simulink model "test4"  (R2024a)
settings: Solver=FixedStepAuto  StartTime=0.0  StopTime=10  FixedStep=0.001  MaxStep=1e-2  RelTol=1e-3
values from neighbouring files (symbols this model uses):
  Current_Torque_ratio = -10.0    [test4.sldd]
  Sigmoid_Range = 2.0    [test4.sldd]
  Simple_HZ = 10.0    [test4.sldd]
libraries: fl_lib x12, nesl_utility x10, sdl_lib x4, slpidlib x3, simulink x2
settings Model: DataDictionary=test4.sldd  Creator=18311  LastModifiedBy=18311

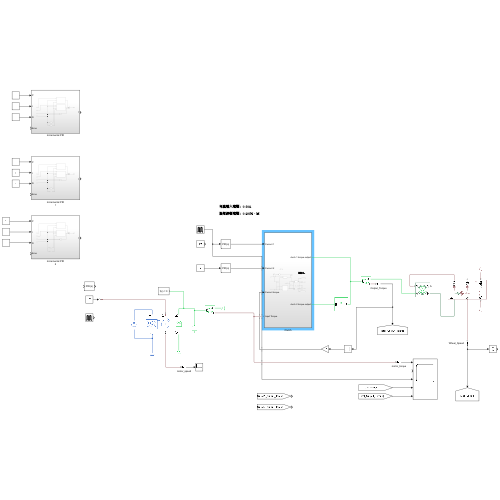
[thumbnail: Simulink's stored preview of the top-level diagram]
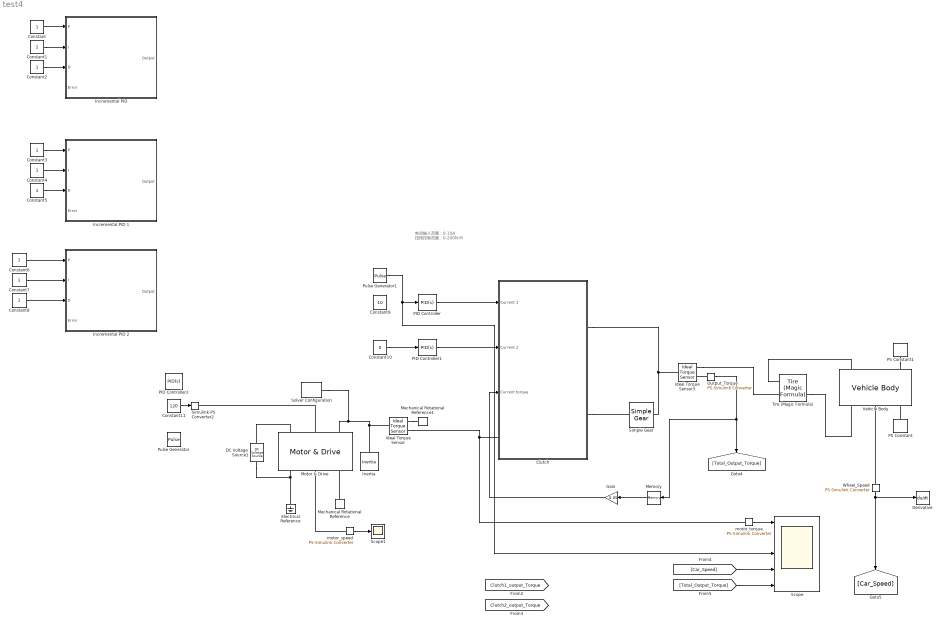
== system test4 ==
  note: 电流输入范围：0-10A
      | 扭矩控制范围：0-200N·M
  Clutch : Subsystem
  Constant{,1..8} (9 alike) : Constant
  Constant10 : Constant  Value=0
  Constant11 : Constant  Value=120
  Constant9 : Constant  Value=10
  DC Voltage Source1 : fl_lib/Electrical/Electrical Sources/DC Voltage Source  v0=220 V
  Derivative : Derivative
  Electrical Reference : fl_lib/Electrical/Electrical Elements/Electrical Reference
  Gain : Gain  Gain=0.05
  Ideal Torque Sensor : fl_lib/Mechanical/Mechanical Sensors/Ideal Torque Sensor
  Ideal Torque Sensor3 : fl_lib/Mechanical/Mechanical Sensors/Ideal Torque Sensor
  "Incremental PID " : Subsystem
  Incremental PID 1 : Subsystem
  Incremental PID 2 : Subsystem
  Inertia : fl_lib/Mechanical/Rotational Elements/Inertia  inertia=0.01 kg*m^2  num_ports=foundation.enum.numPorts2.one  w_specify=off  w_priority=High  w=0 rad/s  w_nominal_specify=off  w_nominal_value=1  w_nominal_unit=rad/s  t_specify=off  t_priority=None  t=0 N*m  t_nominal_specify=off  t_nominal_value=1  t_nominal_unit=N*m
  Mechanical Rotational Reference : fl_lib/Mechanical/Rotational Elements/Mechanical Rotational Reference
  Mechanical Rotational Reference1 : fl_lib/Mechanical/Rotational Elements/Mechanical Rotational Reference
  Memory : Memory
  Motor & Drive : sdl_lib/Engines & Motors/Motor & Drive  torque_max=150 N*m  power_max=20 kW  Tc=1 s  eff=75  w_eff=100 rpm  T_eff=400 N*m  thermal_port=simscape.enum.thermaleffects.omit  thermal_mass=100 J/K  temperature_specify=off  temperature_priority=High  temperature=300 K  temperature_nominal_specify=off  temperature_nominal_value=1  temperature_nominal_unit=K
      settings: InternalSimscapePortConfiguration="{\"Bottom\":[],\"Left\":[{\"id\":\"Vp\",\"label\":\"+\",\"type\":\"foundation.electrical.electrical\"},{\"id\":\"Tr\",\"label\":\"Tr\",\"type\":\"input\"},{\"id\":\"R\",\"label\":\"R\",\"type\":\"foundation.mechanical.rotational.rotational\"}],\"Right\":[{\"id\":\"Vm\",\"label\":\"-\",\"type\":\"foundation.electrical.electrical\"},{\"id\":\"Omega\",\"label\":\"w\",\"type\":\"output\"},{\"id\":\"C\",\"label\":\"C\",\"type\":\"foundation.mechanical.rotational.rotational\"}],\"Top\":[]}"
  Output_Torque : nesl_utility/PS-Simulink Converter  PhysicalDomain=network_engine_domain  SubClassName=ps_output  LeftPortType=input  RightPortType=output  PseudoPeriodic=off  Frequencies=[]  VectorFormat=inherit  Unit=inherit  AffineConversion=off
  PID Controller : slpidlib/PID Controller  Controller=PID  Form=Parallel  TimeDomain=Continuous-time  UseExternalTs=off  SampleTime=-1  IntegratorMethod=Forward Euler  FilterMethod=Forward Euler  ControllerParametersSource=internal  P=1  I=0  UseKiTs=off  D=0  UseExternalDerivativeSource=off  N=100  UseFilter=on  TunerSelectOption=Transfer Function Based (PID Tuner App)  InitialConditionSource=internal  InitialConditionForIntegrator=0  InitialConditionForFilter=0  DifferentiatorICPrevScaledInput=0  ExternalReset=none  TrackingMode=off  Kt=1  LimitOutput=off  SatLimitsSource=internal  UpperSaturationLimit=inf  LowerSaturationLimit=-inf  LinearizeAsGain=on  AntiWindupMode=none  Kb=1  LimitIntegrator=off  UpperIntegratorSaturationLimit=inf  LowerIntegratorSaturationLimit=-inf  POutMin=[]  POutMax=[]  IOutMin=[]  IOutMax=[]  DOutMin=[]  DOutMax=[]  NOutMin=[]  NOutMax=[]  SumOutMin=[]  SumOutMax=[]  SaturationOutMin=[]  SaturationOutMax=[]  PParamMin=[]  PParamMax=[]  IParamMin=[]  IParamMax=[]  DParamMin=[]  DParamMax=[]  NParamMin=[]  NParamMax=[]  KbParamMin=[]  KbParamMax=[]  KtParamMin=[]  KtParamMax=[]  KbOutMin=[]  KbOutMax=[]  KtOutMin=[]  KtOutMax=[]  IntegratorOutMin=[]  IntegratorOutMax=[]  FilterOutMin=[]  FilterOutMax=[]  SumI1OutMin=[]  SumI1OutMax=[]  SumI2OutMin=[]  SumI2OutMax=[]  SumI3OutMin=[]  SumI3OutMax=[]  SumI4OutMin=[]  SumI4OutMax=[]  SumDOutMin=[]  SumDOutMax=[]  DifferentiatorOutMin=[]  DifferentiatorOutMax=[]  FilterDiffOutCoefMin=[]  FilterDiffOutCoefMax=[]  ReciprocalOutMin=[]  ReciprocalOutMax=[]  SumDenOutMin=[]  SumDenOutMax=[]  SumNumOutMin=[]  SumNumOutMax=[]  DivideOutMin=[]  DivideOutMax=[]  UdiffTsProdOutMin=[]  UdiffTsProdOutMax=[]  NTsProdOutMin=[]  NTsProdOutMax=[]  UintegralTsProdOutMin=[]  UintegralTsProdOutMax=[]  UngainTsProdOutMin=[]  UngainTsProdOutMax=[]  ClampingZeroOutDataTypeStr=Inherit: Inherit via back propagation  ClampingZeroOutMin=[]  ClampingZeroOutMax=[]  FilterDenConstantOutDataTypeStr=Inherit: Inherit via back propagation  FilterDenConstantOutMin=[]  FilterDenConstantOutMax=[]  PCopyOutDataTypeStr=Inherit: Inherit via back propagation  PCopyOutMin=[]  PCopyOutMax=[]  NCopyOutDataTypeStr=Inherit: Inherit via back propagation  NCopyOutMin=[]  NCopyOutMax=[]  IntegratorContinuousStateAttributes=''  IntegratorStateMustResolveToSignalObject=off  IntegratorRTWStateStorageClass=Auto  FilterContinuousStateAttributes=''  FilterStateMustResolveToSignalObject=off  FilterRTWStateStorageClass=Auto  ParallelPVariant=InternalParameters  IdealPVariant=Disabled  IVariant=InternalParameters  DVariant=InternalParameters  IntegratorVariant=Continuous  SatVariant=Disabled  AWVariant=Passthrough  PCopyVariant=Disabled  TRVariant=Disabled  FdbkBlocksVariant=Forward  IdealPFdbkVariant=Disabled  SatFdbkVariant=Disabled  DerivativeFilterVariant=ContFilter  NVariant=InternalParameters  NCopyVariant=Disabled  FilterICVariant=InternalICsFilter  IntegratorICVariant=InternalICs  ExternalResetVariant=Disabled  TRSumVariant=Passthrough  SumFdbkVariant=Disabled  SumVariant=Sum_PID  TsampFilterVariant=InternalTs  TsampNgainVariant=Passthrough  TsampIntegralVariant=Disabled_SignalSpec  ExternalSaturationOutDataTypeStr=Inherit: Same as second input  DerivativeSourceVariant=ErrorSignal
  PID Controller1 : slpidlib/PID Controller  Controller=PID  Form=Parallel  TimeDomain=Continuous-time  UseExternalTs=off  SampleTime=-1  IntegratorMethod=Forward Euler  FilterMethod=Forward Euler  ControllerParametersSource=internal  P=1  I=0  UseKiTs=off  D=0  UseExternalDerivativeSource=off  N=100  UseFilter=on  TunerSelectOption=Transfer Function Based (PID Tuner App)  InitialConditionSource=internal  InitialConditionForIntegrator=0  InitialConditionForFilter=0  DifferentiatorICPrevScaledInput=0  ExternalReset=none  TrackingMode=off  Kt=1  LimitOutput=off  SatLimitsSource=internal  UpperSaturationLimit=inf  LowerSaturationLimit=-inf  LinearizeAsGain=on  AntiWindupMode=none  Kb=1  LimitIntegrator=off  UpperIntegratorSaturationLimit=inf  LowerIntegratorSaturationLimit=-inf  POutMin=[]  POutMax=[]  IOutMin=[]  IOutMax=[]  DOutMin=[]  DOutMax=[]  NOutMin=[]  NOutMax=[]  SumOutMin=[]  SumOutMax=[]  SaturationOutMin=[]  SaturationOutMax=[]  PParamMin=[]  PParamMax=[]  IParamMin=[]  IParamMax=[]  DParamMin=[]  DParamMax=[]  NParamMin=[]  NParamMax=[]  KbParamMin=[]  KbParamMax=[]  KtParamMin=[]  KtParamMax=[]  KbOutMin=[]  KbOutMax=[]  KtOutMin=[]  KtOutMax=[]  IntegratorOutMin=[]  IntegratorOutMax=[]  FilterOutMin=[]  FilterOutMax=[]  SumI1OutMin=[]  SumI1OutMax=[]  SumI2OutMin=[]  SumI2OutMax=[]  SumI3OutMin=[]  SumI3OutMax=[]  SumI4OutMin=[]  SumI4OutMax=[]  SumDOutMin=[]  SumDOutMax=[]  DifferentiatorOutMin=[]  DifferentiatorOutMax=[]  FilterDiffOutCoefMin=[]  FilterDiffOutCoefMax=[]  ReciprocalOutMin=[]  ReciprocalOutMax=[]  SumDenOutMin=[]  SumDenOutMax=[]  SumNumOutMin=[]  SumNumOutMax=[]  DivideOutMin=[]  DivideOutMax=[]  UdiffTsProdOutMin=[]  UdiffTsProdOutMax=[]  NTsProdOutMin=[]  NTsProdOutMax=[]  UintegralTsProdOutMin=[]  UintegralTsProdOutMax=[]  UngainTsProdOutMin=[]  UngainTsProdOutMax=[]  ClampingZeroOutDataTypeStr=Inherit: Inherit via back propagation  ClampingZeroOutMin=[]  ClampingZeroOutMax=[]  FilterDenConstantOutDataTypeStr=Inherit: Inherit via back propagation  FilterDenConstantOutMin=[]  FilterDenConstantOutMax=[]  PCopyOutDataTypeStr=Inherit: Inherit via back propagation  PCopyOutMin=[]  PCopyOutMax=[]  NCopyOutDataTypeStr=Inherit: Inherit via back propagation  NCopyOutMin=[]  NCopyOutMax=[]  IntegratorContinuousStateAttributes=''  IntegratorStateMustResolveToSignalObject=off  IntegratorRTWStateStorageClass=Auto  FilterContinuousStateAttributes=''  FilterStateMustResolveToSignalObject=off  FilterRTWStateStorageClass=Auto  ParallelPVariant=InternalParameters  IdealPVariant=Disabled  IVariant=InternalParameters  DVariant=InternalParameters  IntegratorVariant=Continuous  SatVariant=Disabled  AWVariant=Passthrough  PCopyVariant=Disabled  TRVariant=Disabled  FdbkBlocksVariant=Forward  IdealPFdbkVariant=Disabled  SatFdbkVariant=Disabled  DerivativeFilterVariant=ContFilter  NVariant=InternalParameters  NCopyVariant=Disabled  FilterICVariant=InternalICsFilter  IntegratorICVariant=InternalICs  ExternalResetVariant=Disabled  TRSumVariant=Passthrough  SumFdbkVariant=Disabled  SumVariant=Sum_PID  TsampFilterVariant=InternalTs  TsampNgainVariant=Passthrough  TsampIntegralVariant=Disabled_SignalSpec  ExternalSaturationOutDataTypeStr=Inherit: Same as second input  DerivativeSourceVariant=ErrorSignal
  PID Controller2 : slpidlib/PID Controller  Controller=PID  Form=Parallel  TimeDomain=Continuous-time  UseExternalTs=off  SampleTime=-1  IntegratorMethod=Forward Euler  FilterMethod=Forward Euler  ControllerParametersSource=internal  P=1  I=1  UseKiTs=off  D=0  UseExternalDerivativeSource=off  N=100  UseFilter=on  TunerSelectOption=Transfer Function Based (PID Tuner App)  InitialConditionSource=internal  InitialConditionForIntegrator=0  InitialConditionForFilter=0  DifferentiatorICPrevScaledInput=0  ExternalReset=none  TrackingMode=off  Kt=1  LimitOutput=off  SatLimitsSource=internal  UpperSaturationLimit=inf  LowerSaturationLimit=-inf  LinearizeAsGain=on  AntiWindupMode=none  Kb=1  LimitIntegrator=off  UpperIntegratorSaturationLimit=inf  LowerIntegratorSaturationLimit=-inf  POutMin=[]  POutMax=[]  IOutMin=[]  IOutMax=[]  DOutMin=[]  DOutMax=[]  NOutMin=[]  NOutMax=[]  SumOutMin=[]  SumOutMax=[]  SaturationOutMin=[]  SaturationOutMax=[]  PParamMin=[]  PParamMax=[]  IParamMin=[]  IParamMax=[]  DParamMin=[]  DParamMax=[]  NParamMin=[]  NParamMax=[]  KbParamMin=[]  KbParamMax=[]  KtParamMin=[]  KtParamMax=[]  KbOutMin=[]  KbOutMax=[]  KtOutMin=[]  KtOutMax=[]  IntegratorOutMin=[]  IntegratorOutMax=[]  FilterOutMin=[]  FilterOutMax=[]  SumI1OutMin=[]  SumI1OutMax=[]  SumI2OutMin=[]  SumI2OutMax=[]  SumI3OutMin=[]  SumI3OutMax=[]  SumI4OutMin=[]  SumI4OutMax=[]  SumDOutMin=[]  SumDOutMax=[]  DifferentiatorOutMin=[]  DifferentiatorOutMax=[]  FilterDiffOutCoefMin=[]  FilterDiffOutCoefMax=[]  ReciprocalOutMin=[]  ReciprocalOutMax=[]  SumDenOutMin=[]  SumDenOutMax=[]  SumNumOutMin=[]  SumNumOutMax=[]  DivideOutMin=[]  DivideOutMax=[]  UdiffTsProdOutMin=[]  UdiffTsProdOutMax=[]  NTsProdOutMin=[]  NTsProdOutMax=[]  UintegralTsProdOutMin=[]  UintegralTsProdOutMax=[]  UngainTsProdOutMin=[]  UngainTsProdOutMax=[]  ClampingZeroOutDataTypeStr=Inherit: Inherit via back propagation  ClampingZeroOutMin=[]  ClampingZeroOutMax=[]  FilterDenConstantOutDataTypeStr=Inherit: Inherit via back propagation  FilterDenConstantOutMin=[]  FilterDenConstantOutMax=[]  PCopyOutDataTypeStr=Inherit: Inherit via back propagation  PCopyOutMin=[]  PCopyOutMax=[]  NCopyOutDataTypeStr=Inherit: Inherit via back propagation  NCopyOutMin=[]  NCopyOutMax=[]  IntegratorContinuousStateAttributes=''  IntegratorStateMustResolveToSignalObject=off  IntegratorRTWStateStorageClass=Auto  FilterContinuousStateAttributes=''  FilterStateMustResolveToSignalObject=off  FilterRTWStateStorageClass=Auto  ParallelPVariant=InternalParameters  IdealPVariant=Disabled  IVariant=InternalParameters  DVariant=InternalParameters  IntegratorVariant=Continuous  SatVariant=Disabled  AWVariant=Passthrough  PCopyVariant=Disabled  TRVariant=Disabled  FdbkBlocksVariant=Forward  IdealPFdbkVariant=Disabled  SatFdbkVariant=Disabled  DerivativeFilterVariant=ContFilter  NVariant=InternalParameters  NCopyVariant=Disabled  FilterICVariant=InternalICsFilter  IntegratorICVariant=InternalICs  ExternalResetVariant=Disabled  TRSumVariant=Passthrough  SumFdbkVariant=Disabled  SumVariant=Sum_PID  TsampFilterVariant=InternalTs  TsampNgainVariant=Passthrough  TsampIntegralVariant=Disabled_SignalSpec  ExternalSaturationOutDataTypeStr=Inherit: Same as second input  DerivativeSourceVariant=ErrorSignal
  PS Constant : fl_lib/Physical Signals/Sources/PS Constant  constant=0
  PS Constant1 : fl_lib/Physical Signals/Sources/PS Constant  constant=0
  Pulse Generator : DiscretePulseGenerator  PulseType=Time based  Amplitude=50  Period=50  PulseWidth=50
  Pulse Generator1 : DiscretePulseGenerator  PulseType=Time based  Amplitude=10  Period=10  PulseWidth=50  PhaseDelay=2
  Scope : Scope  NumInputPorts=5
  Scope1 : Scope
  Simple Gear : sdl_lib/Gears/Simple Gear  ratio=3  rotation_direction=sdl.enum.shaftOutputDirection.same  enable_faults=simscape.enum.onoff.off  efficiency_fault=0.05  fault_angles=pi / 12 rad  friction_model=sdl.enum.gear_efficiencies_load.off  T_noload=0.1 N*m  T_nom=5 N*m  efficiency_nom=0.8  efficiency=0.8  temperature_TLU=[280, 300, 320] K  load_TLU=[1, 5, 10] N*m  efficiency_TLU=[.95, .9, .85]  efficiency_TLU2=[.85, .8, .75; .95, .9, .85; .85, .8, .7]  w_thr=0.01 rad/s  pwr_thr=0.001 W  enable_backlash=false  hardstop_model=simscape.enum.hardstop.smooth  backlash_distance=1e-3 mm  r_base=0.1 m  transition=1e-4 mm  backlash_stiffness=1e6 N/m  backlash_damping=1e3 N*s/m  coeff_rest=0.7  v_tol=0.001 m/s  f_tol=0.001 N  mu_visc=[0, 0] N*m*s/rad  thermal_mass=50 J/K  temperature_specify=off  temperature_priority=High  temperature=300 K  temperature_nominal_specify=off  temperature_nominal_value=1  temperature_nominal_unit=K  x_backlash_specify=off  x_backlash_priority=None  x_backlash=0 mm  x_backlash_nominal_specify=off  x_backlash_nominal_value=1  x_backlash_nominal_unit=mm  f_hardstop_specify=off  f_hardstop_priority=None  f_hardstop=0 N  f_hardstop_nominal_specify=off  f_hardstop_nominal_value=1  f_hardstop_nominal_unit=N  v_backlash_specify=off  v_backlash_priority=None  v_backlash=0 m/s  v_backlash_nominal_specify=off  v_backlash_nominal_value=1  v_backlash_nominal_unit=m/s
  Simulink-PS Converter2 : nesl_utility/Simulink-PS Converter  PhysicalDomain=network_engine_domain  SubClassName=ps_input  LeftPortType=input  RightPortType=output  PseudoPeriodic=off  Frequencies=[]  NoiseDistribution=none  NoiseParameters=[]  Unit=1  AffineConversion=off  FilteringAndDerivatives=provide  SimscapeFilterOrder=1  InputFilterTimeConstant=0.001  UdotUserProvided=0
  Solver Configuration : nesl_utility/Solver Configuration  PhysicalDomain=network_engine_domain  SubClassName=solver  LeftPortType=input  RightPortType=generic  Tones=[]  Harmonics=[]  SimulateNoise=off  Profile=off  UseLocalSampling=off  EnableSwitchedLinearOptims=on  FrequencyDomain=off  UseCCode=off  RelTol=0.001  AbsTol=0.001  MinStep=1e-09  ToWorkspace=off  RevertToSquareIcSolve=off  NumHomotopyIterations=100  PhasorMode=off  PhasorModeNumHarmonics=1  ConsistencySolver=NEWTON_XTOL_AFTER_FTOL  IndexReductionMethod=DerivativeReplacement  DoDC=off  ResidualTolerance=1e-09  ConsistencyTolSource=GLOBAL  ConsistencyAbsTol=0.001  ConsistencyRelTol=0.001  ConsistencyTolFactor=0.001  UseLocalSolver=off  LocalSolverChoice=NE_BACKWARD_EULER_ADVANCER  ResolveIndetEquations=on  FunctionEvalNumThread=1  LocalSolverSampleTime=0.001  DoFixedCost=off  MaxNonlinIter=3  MaxModeIter=2  ComputeImpulses=off  ImpulseIterations=2  LinearAlgebra=auto  LinearAlgebraNumThread=0  EquationFormulation=NE_TIME_EF  DelaysMemoryBudget=1024  AutomaticFiltering=on  FilteringTimeConstant=0.001  PartitionStorageMethod=AS_NEEDED  PartitionMemoryBudget=1024  PartitionMethod=ROBUST  MultibodyUseLocalSolver=off  MultibodyLocalSolverChoice=ODE1  MultibodyLocalSolverSampleTime=0.001
  Tire (Magic Formula) : sdl_lib/Tires & Vehicles/Tire (Magic Formula)  parameterization=sdl.enum.magic_tire_model.peak  F_z1=3000 N  F_x1=3500 N  kappa1=10  B_m=10  C_m=1.9  D_m=1  E_m=0.97  fz0=4000 N  p_Cx=1.685  p_Dx=[1.21, -.037]  p_Ex=[.344, .095, -.02, 0]  p_Kx=[21.51, -.163, .245]  p_Hx=[-.002, .002]  p_Vx=[0, 0]  rolling_radius_model=sdl.enum.RollingRadiusParameterization.Constant  r_e=0.3 m  r_0=0.3 m  breff=8.39  dreff=0.26  freff=0.074  q_re0=0.99  q_v1=0.008  longvl=17 m/s  cz=5e5 N/m  model_resistance=false  resistance_model=sdl.enum.rollingResistanceParameterization.constant  coeff=0.015  p_tire=250e3 Pa  alpha=-0.003  beta=0.97  coeff_a=84e-4  coeff_b=6.2e-4 s/m  coeff_c=1.6e-4 s^2/m^2  p_tire0=240e3 Pa  fz0_resistance=4000 N  vH0=16 m/s  q_Sy=[.0082, 0, .0014, .001, 0, 0, 1.08, -.5]  v_thr=0.001 m/s  enable_scaling_coefficients=false  lfzO=1  lcx=1  lmux=1  lex=1  lkx=1  lhx=1  lvx=1  lmy=1  model_compliance=sdl.enum.compliance.off  stiffness=1e6 N/m  damping=1000 N*s/m  model_inertia=sdl.enum.model_inertia.off  inertia=1 kg*m^2  initial_velocity=0 rad/s  vxlow=1 m/s  v_tr_thr=0.1 m/s  kpumin=-1.5  kpumax=1.5
  Vehicle Body : sdl_lib/Tires & Vehicles/Vehicle Body  mass=1200 kg  n_w=2  x_f=1.4 m  x_r=1.6 m  y_c=0.5 m  mass_var=simscape.enum.onoff.off  g=9.81 m/s^2  liftoff_warning=simscape.enum.onoff.off  area=3 m^2  Cd=0.4  rho=1.18 kg/m^3  model_pitch=simscape.enum.onoff.off  inertia=4000 kg*m^2  suspension_model=sdl.enum.linearTLU.linear  k_f=1e4 N/m  b_f=1e4 N*s/m  k_r=1e4 N/m  b_r=1e4 N*s/m  k_f_TLU=[-2000, -1000, 0, 1000, 2000] N  x_f_TLU=[-.4, -.2, 0, .2, .4] m  b_f_TLU=[-200, -100, 0, 100, 200] N  v_f_TLU=[-4, -2, 0, 2, 4] m/s  k_r_TLU=[-2000, -1000, 0, 1000, 2000] N  x_r_TLU=[-.4, -.2, 0, .2, .4] m  b_r_TLU=[-200, -100, 0, 100, 200] N  v_r_TLU=[-4, -2, 0, 2, 4] m/s  interp_method=simscape.enum.interpolation.linear  extrap_method=simscape.enum.extrapolation.linear  model_hardstop=simscape.enum.onoff.off  upper_bound_f=.25 m  lower_bound_f=-.25 m  stop_k_f=1e6 N/m  stop_b_f=150 N*s/m  upper_bound_r=.25 m  lower_bound_r=-.25 m  stop_k_r=1e6 N/m  stop_b_r=150 N*s/m  initial_pitch=0 rad  initial_pitch_rate=0 rad/s  v_specify=off  v_priority=High  v=0 m/s  v_nominal_specify=off  v_nominal_value=1  v_nominal_unit=m/s
  Wheel_Speed : nesl_utility/PS-Simulink Converter  PhysicalDomain=network_engine_domain  SubClassName=ps_output  LeftPortType=input  RightPortType=output  PseudoPeriodic=off  Frequencies=[]  VectorFormat=inherit  Unit=inherit  AffineConversion=off
  motor_speed : nesl_utility/PS-Simulink Converter  PhysicalDomain=network_engine_domain  SubClassName=ps_output  LeftPortType=input  RightPortType=output  PseudoPeriodic=off  Frequencies=[]  VectorFormat=inherit  Unit=inherit  AffineConversion=off
  motor_torque : nesl_utility/PS-Simulink Converter  PhysicalDomain=network_engine_domain  SubClassName=ps_output  LeftPortType=input  RightPortType=output  PseudoPeriodic=off  Frequencies=[]  VectorFormat=inherit  Unit=inherit  AffineConversion=off
  wires:
  motor_torque/1 -> Scope/1
  motor_speed/1 -> Scope1/1
  Wheel_Speed/1 -> [Car_Speed], Derivative/1
  Gain/1 -> Clutch/3(Current torque)
  Constant/1 -> "Incremental PID "/1(P)
  Constant1/1 -> "Incremental PID "/2(I)
  Constant2/1 -> "Incremental PID "/3(D)
  Constant3/1 -> Incremental PID 1/1(P)
  Constant4/1 -> Incremental PID 1/2(I)
  Constant5/1 -> Incremental PID 1/3(D)
  Constant6/1 -> Incremental PID 2/1(P)
  Constant7/1 -> Incremental PID 2/2(I)
  Constant8/1 -> Incremental PID 2/3(D)
  PID Controller/1 -> Clutch/1(Current 1)
  PID Controller1/1 -> Clutch/2(Current 2)
  Constant10/1 -> PID Controller1/1
  Constant11/1 -> Simulink-PS Converter2/1
  [Total_Output_Torque] -> Scope/5
  [Car_Speed] -> Scope/4
  Pulse Generator1/1 -> PID Controller/1, Scope/3
  Memory/1 -> Gain/1
  Output_Torque/1 -> Memory/1, [Total_Output_Torque]
  connections:
  Motor & Drive/LConn1 -- DC Voltage Source1/LConn1
  Electrical Reference/LConn1 -- DC Voltage Source1/RConn1 -- Motor & Drive/RConn1
  Mechanical Rotational Reference/LConn1 -- Motor & Drive/RConn3
  Inertia/LConn1 -- Solver Configuration/RConn1 -- Motor & Drive/LConn3 -- Ideal Torque Sensor/LConn1
  Tire (Magic Formula)/RConn2 -- Vehicle Body/LConn1
  Vehicle Body/RConn1 -- Tire (Magic Formula)/LConn1
  PS Constant/RConn1 -- Vehicle Body/LConn3
  PS Constant1/RConn1 -- Vehicle Body/RConn3
  Ideal Torque Sensor3/LConn1 -- Simple Gear/RConn1 -- Clutch/RConn1
  Ideal Torque Sensor/RConn2 -- Clutch/LConn1 -- motor_torque/LConn1
  Wheel_Speed/LConn1 -- Vehicle Body/LConn2
  motor_speed/LConn1 -- Motor & Drive/RConn2
  Ideal Torque Sensor3/RConn1 -- Tire (Magic Formula)/LConn2
  Output_Torque/LConn1 -- Ideal Torque Sensor3/RConn2
  Ideal Torque Sensor/RConn1 -- Mechanical Rotational Reference1/LConn1
  Clutch/RConn2 -- Simple Gear/LConn1
  Motor & Drive/LConn2 -- Simulink-PS Converter2/RConn1

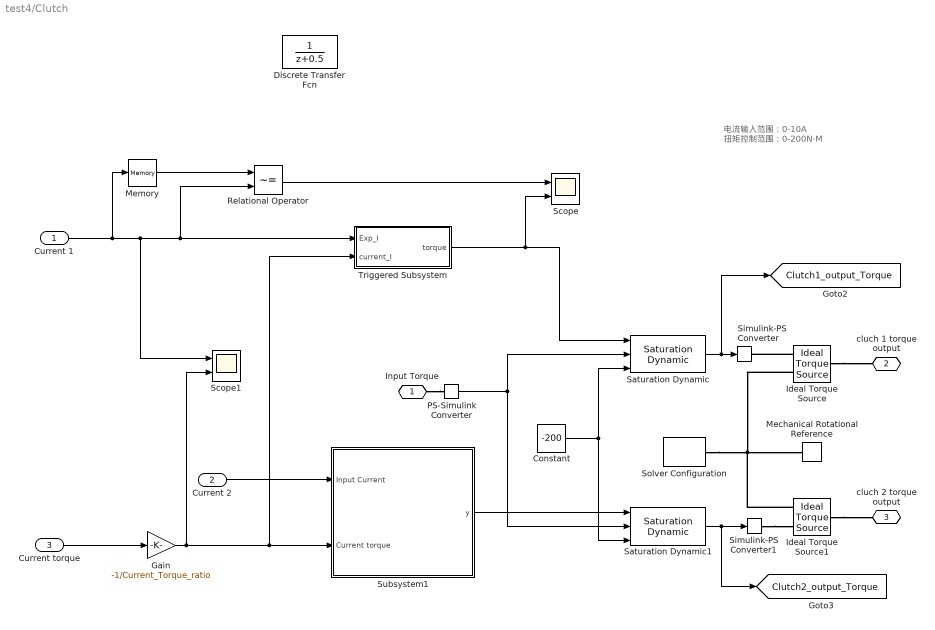
== system test4/Clutch ==
  note: 电流输入范围：0-10A
      | 扭矩控制范围：0-200N·M
  Current 1 : Inport
  Current 2 : Inport  Port=2
  Current torque : Inport  Port=3
  Constant : Constant  Value=-200
  Discrete Transfer Fcn : DiscreteTransferFcn
  Gain : Gain  Gain=-1/Current_Torque_ratio
  Ideal Torque Source : fl_lib/Mechanical/Mechanical Sources/Ideal Torque Source
  Ideal Torque Source1 : fl_lib/Mechanical/Mechanical Sources/Ideal Torque Source
  Mechanical Rotational Reference : fl_lib/Mechanical/Rotational Elements/Mechanical Rotational Reference
  Memory : Memory
  PS-Simulink Converter : nesl_utility/PS-Simulink Converter  PhysicalDomain=network_engine_domain  SubClassName=ps_output  LeftPortType=input  RightPortType=output  PseudoPeriodic=off  Frequencies=[]  VectorFormat=inherit  Unit=inherit  AffineConversion=off
  Relational Operator : RelationalOperator  Operator=~=  OutDataTypeStr=boolean  RndMeth=Simplest  InputSameDT=off
  Saturation Dynamic : simulink/Discontinuities/Saturation Dynamic  OutMin=[]  OutMax=[]  OutDataTypeStr=Inherit: Same as second input  OutDataType=fixdt(1, 16)  OutScaling=2^-10  DoSatur=off
  Saturation Dynamic1 : simulink/Discontinuities/Saturation Dynamic  OutMin=[]  OutMax=[]  OutDataTypeStr=Inherit: Same as second input  OutDataType=fixdt(1, 16)  OutScaling=2^-10  DoSatur=off
  Scope : Scope  NumInputPorts=2
  Scope1 : Scope  NumInputPorts=2
  Simulink-PS Converter : nesl_utility/Simulink-PS Converter  PhysicalDomain=network_engine_domain  SubClassName=ps_input  LeftPortType=input  RightPortType=output  PseudoPeriodic=off  Frequencies=[]  NoiseDistribution=none  NoiseParameters=[]  Unit=1  AffineConversion=off  FilteringAndDerivatives=provide  SimscapeFilterOrder=1  InputFilterTimeConstant=0.001  UdotUserProvided=0
  Simulink-PS Converter1 : nesl_utility/Simulink-PS Converter  PhysicalDomain=network_engine_domain  SubClassName=ps_input  LeftPortType=input  RightPortType=output  PseudoPeriodic=off  Frequencies=[]  NoiseDistribution=none  NoiseParameters=[]  Unit=1  AffineConversion=off  FilteringAndDerivatives=provide  SimscapeFilterOrder=1  InputFilterTimeConstant=0.001  UdotUserProvided=0
  Solver Configuration : nesl_utility/Solver Configuration  PhysicalDomain=network_engine_domain  SubClassName=solver  LeftPortType=input  RightPortType=generic  Tones=[]  Harmonics=[]  SimulateNoise=off  Profile=off  UseLocalSampling=off  EnableSwitchedLinearOptims=on  FrequencyDomain=off  UseCCode=off  RelTol=0.001  AbsTol=0.001  MinStep=1e-09  ToWorkspace=off  RevertToSquareIcSolve=off  NumHomotopyIterations=100  PhasorMode=off  PhasorModeNumHarmonics=1  ConsistencySolver=NEWTON_XTOL_AFTER_FTOL  IndexReductionMethod=DerivativeReplacement  DoDC=off  ResidualTolerance=1e-09  ConsistencyTolSource=GLOBAL  ConsistencyAbsTol=0.001  ConsistencyRelTol=0.001  ConsistencyTolFactor=0.001  UseLocalSolver=off  LocalSolverChoice=NE_BACKWARD_EULER_ADVANCER  ResolveIndetEquations=on  FunctionEvalNumThread=1  LocalSolverSampleTime=0.001  DoFixedCost=off  MaxNonlinIter=3  MaxModeIter=2  ComputeImpulses=off  ImpulseIterations=2  LinearAlgebra=auto  LinearAlgebraNumThread=0  EquationFormulation=NE_TIME_EF  DelaysMemoryBudget=1024  AutomaticFiltering=on  FilteringTimeConstant=0.001  PartitionStorageMethod=AS_NEEDED  PartitionMemoryBudget=1024  PartitionMethod=ROBUST  MultibodyUseLocalSolver=off  MultibodyLocalSolverChoice=ODE1  MultibodyLocalSolverSampleTime=0.001
  Subsystem1 : Subsystem
  Triggered Subsystem : Subsystem  TreatAsAtomicUnit=on
  Input Torque : PMIOPort  Side=Left
  cluch 1 torque output : PMIOPort  Port=2  Side=Right
  cluch 2 torque output : PMIOPort  Port=3  Side=Right
  tag scope: Clutch1_output_Torque=global, Clutch2_output_Torque=global
  wires:
  Subsystem1/1(y) -> Saturation Dynamic1/1
  Current 2/1 -> Subsystem1/1(Input Current)
  Current torque/1 -> Gain/1
  PS-Simulink Converter/1 -> Saturation Dynamic/2, Saturation Dynamic1/2
  Constant/1 -> Saturation Dynamic/3, Saturation Dynamic1/3
  Saturation Dynamic/1 -> [Clutch1_output_Torque], Simulink-PS Converter/1
  Saturation Dynamic1/1 -> [Clutch2_output_Torque], Simulink-PS Converter1/1
  Current 1/1 -> Memory/1, Scope1/1, Relational Operator/2, Triggered Subsystem/1(Exp_I)
  Triggered Subsystem/1(torque) -> Scope/2, Saturation Dynamic/1
  Memory/1 -> Relational Operator/1
  Relational Operator/1 -> Scope/1
  Gain/1 -> Scope1/2, Triggered Subsystem/2(current_I), Subsystem1/2(Current torque)
  connections:
  Input Torque/RConn1 -- PS-Simulink Converter/LConn1
  Ideal Torque Source/RConn1 -- Simulink-PS Converter/RConn1
  Ideal Torque Source/RConn2 -- Solver Configuration/RConn1 -- Ideal Torque Source1/RConn2 -- Mechanical Rotational Reference/LConn1
  Ideal Torque Source/LConn1 -- cluch 1 torque output/RConn1
  Ideal Torque Source1/LConn1 -- cluch 2 torque output/RConn1
  Simulink-PS Converter1/RConn1 -- Ideal Torque Source1/RConn1

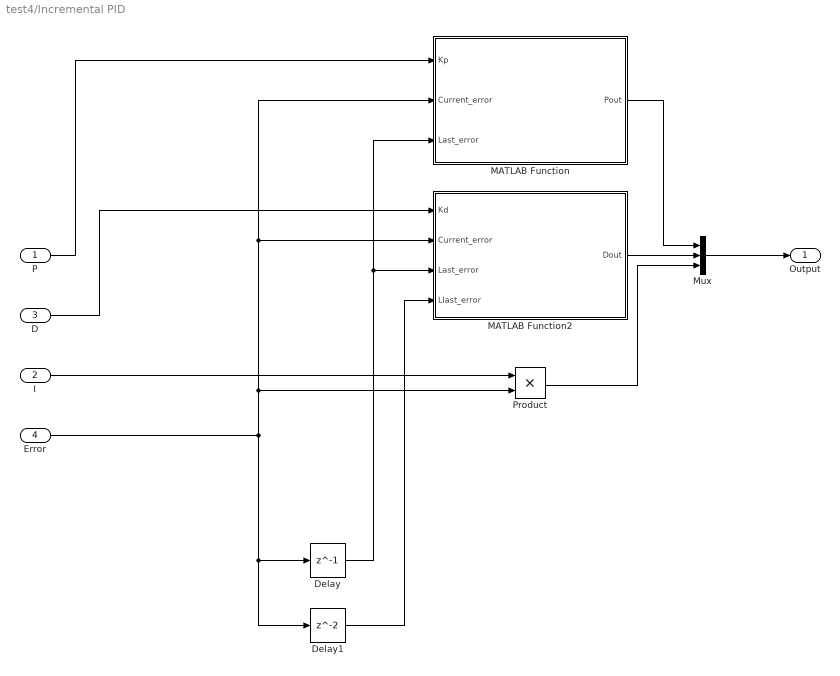
== system test4/Incremental PID  ==
  P : Inport
  I : Inport  Port=2
  D : Inport  Port=3
  Error : Inport  Port=4
  Delay : Delay  DelayLength=1
  Delay1 : Delay
  MATLAB Function : MATLAB Function  TreatAsAtomicUnit=on
  MATLAB Function2 : MATLAB Function  TreatAsAtomicUnit=on
  Mux : Mux  Inputs=3
  Product : Product
  Output : Outport
  wires:
  Error/1 -> MATLAB Function2/2(Current_error), MATLAB Function/2(Current_error), Product/2, Delay1/1, Delay/1
  P/1 -> MATLAB Function/1(Kp)
  D/1 -> MATLAB Function2/1(Kd)
  I/1 -> Product/1
  Product/1 -> Mux/3
  MATLAB Function2/1(Dout) -> Mux/2
  MATLAB Function/1(Pout) -> Mux/1
  Mux/1 -> Output/1
  Delay/1 -> MATLAB Function/3(Last_error), MATLAB Function2/3(Last_error)
  Delay1/1 -> MATLAB Function2/4(Llast_error)

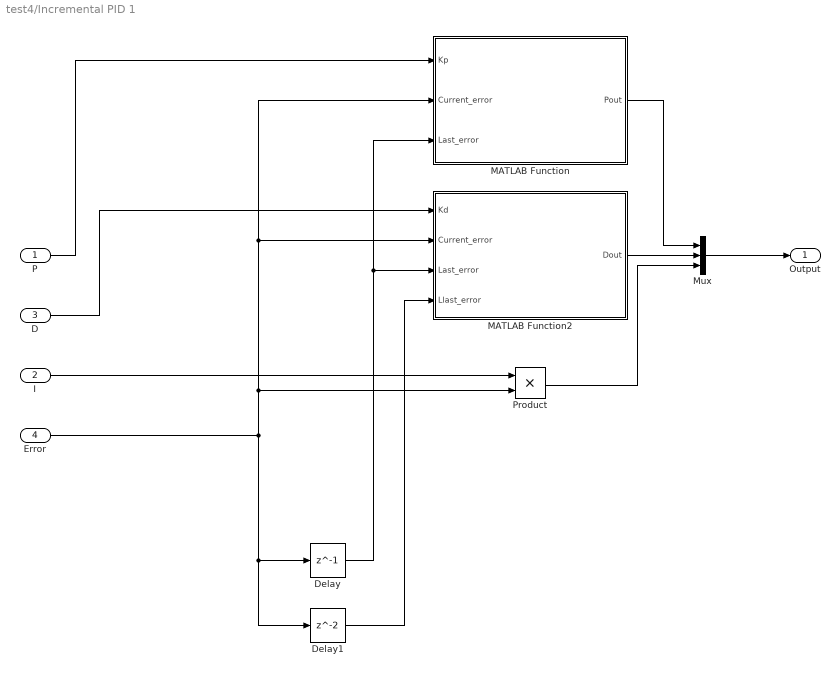
== system test4/Incremental PID 1 ==
  P : Inport
  I : Inport  Port=2
  D : Inport  Port=3
  Error : Inport  Port=4
  Delay : Delay  DelayLength=1
  Delay1 : Delay
  MATLAB Function : MATLAB Function  TreatAsAtomicUnit=on
  MATLAB Function2 : MATLAB Function  TreatAsAtomicUnit=on
  Mux : Mux  Inputs=3
  Product : Product
  Output : Outport
  wires:
  Error/1 -> MATLAB Function2/2(Current_error), MATLAB Function/2(Current_error), Product/2, Delay1/1, Delay/1
  P/1 -> MATLAB Function/1(Kp)
  D/1 -> MATLAB Function2/1(Kd)
  I/1 -> Product/1
  Product/1 -> Mux/3
  MATLAB Function2/1(Dout) -> Mux/2
  MATLAB Function/1(Pout) -> Mux/1
  Mux/1 -> Output/1
  Delay/1 -> MATLAB Function/3(Last_error), MATLAB Function2/3(Last_error)
  Delay1/1 -> MATLAB Function2/4(Llast_error)

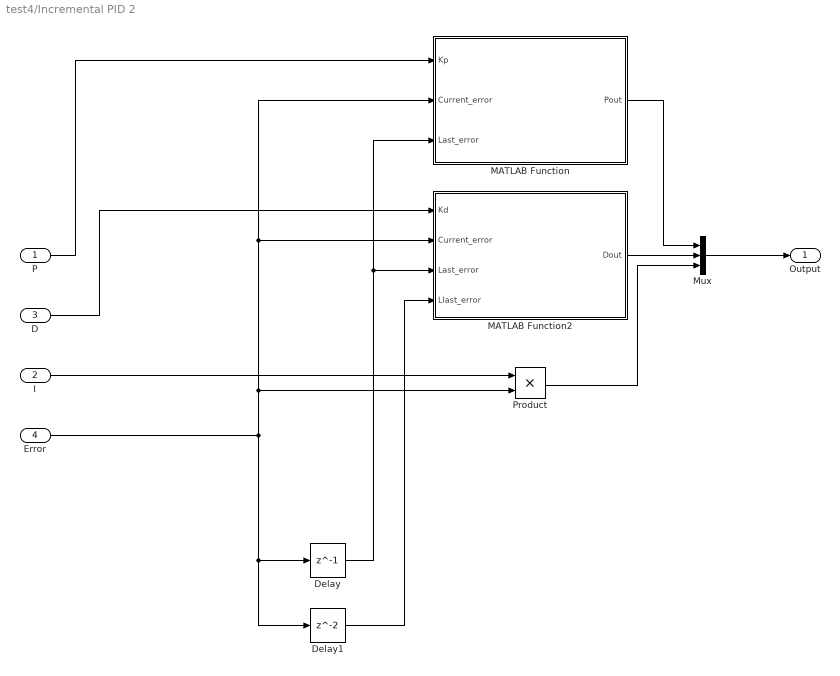
== system test4/Incremental PID 2 ==
  P : Inport
  I : Inport  Port=2
  D : Inport  Port=3
  Error : Inport  Port=4
  Delay : Delay  DelayLength=1
  Delay1 : Delay
  MATLAB Function : MATLAB Function  TreatAsAtomicUnit=on
  MATLAB Function2 : MATLAB Function  TreatAsAtomicUnit=on
  Mux : Mux  Inputs=3
  Product : Product
  Output : Outport
  wires:
  Error/1 -> MATLAB Function2/2(Current_error), MATLAB Function/2(Current_error), Product/2, Delay1/1, Delay/1
  P/1 -> MATLAB Function/1(Kp)
  D/1 -> MATLAB Function2/1(Kd)
  I/1 -> Product/1
  Product/1 -> Mux/3
  MATLAB Function2/1(Dout) -> Mux/2
  MATLAB Function/1(Pout) -> Mux/1
  Mux/1 -> Output/1
  Delay/1 -> MATLAB Function/3(Last_error), MATLAB Function2/3(Last_error)
  Delay1/1 -> MATLAB Function2/4(Llast_error)

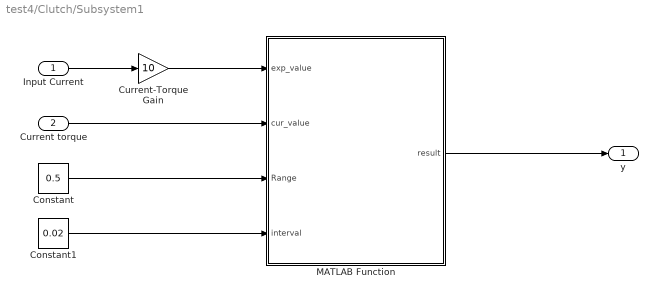
== system test4/Clutch/Subsystem1 ==
  Input Current : Inport
  Current torque : Inport  Port=2
  Constant : Constant  Value=0.5
  Constant1 : Constant  Value=0.02
  Current-Torque Gain : Gain  Gain=10
  MATLAB Function : MATLAB Function  TreatAsAtomicUnit=on
  y : Outport
  wires:
  MATLAB Function/1(result) -> y/1
  Current torque/1 -> MATLAB Function/2(cur_value)
  Input Current/1 -> Current-Torque Gain/1
  Current-Torque Gain/1 -> MATLAB Function/1(exp_value)
  Constant/1 -> MATLAB Function/3(Range)
  Constant1/1 -> MATLAB Function/4(interval)

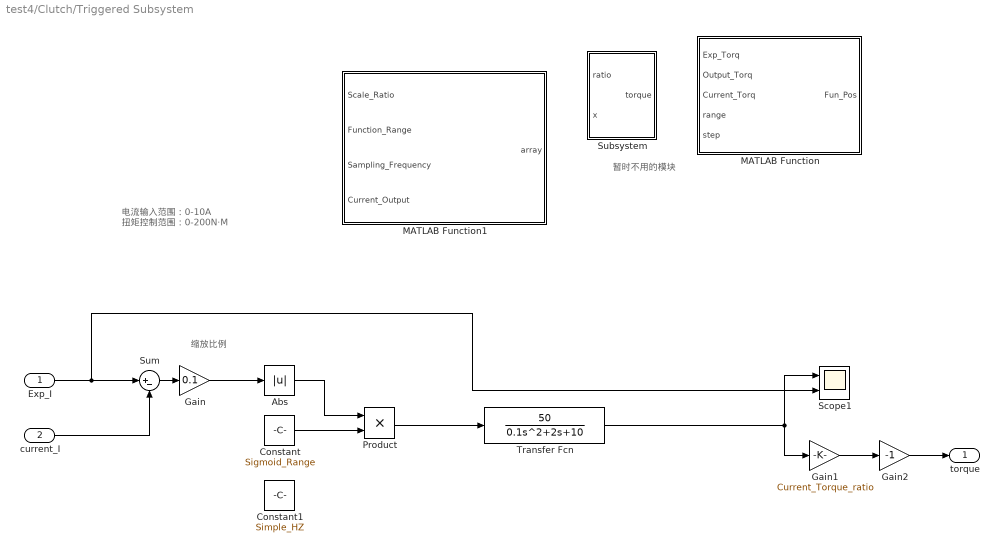
== system test4/Clutch/Triggered Subsystem ==
  note: 暂时不用的模块
  note: 电流输入范围：0-10A
      | 扭矩控制范围：0-200N·M
  note: 缩放比例
  Exp_I : Inport
  current_I : Inport  Port=2
  Abs : Abs  SaturateOnIntegerOverflow=off
  Constant : Constant  Value=Sigmoid_Range
  Constant1 : Constant  Value=Simple_HZ
  Gain : Gain  Gain=0.1
  Gain1 : Gain  Gain=Current_Torque_ratio
  Gain2 : Gain  Gain=-1
  MATLAB Function : MATLAB Function  TreatAsAtomicUnit=on
  MATLAB Function1 : MATLAB Function  TreatAsAtomicUnit=on
  Product : Product
  Scope1 : Scope  NumInputPorts=2
  Subsystem : Subsystem
  Sum : Sum  Inputs=|+-
  Transfer Fcn : TransferFcn  Numerator=[50]  Denominator=[0.1 2 10]
  torque : Outport
  wires:
  Exp_I/1 -> Scope1/2, Sum/1
  Constant/1 -> Product/2
  Abs/1 -> Product/1
  current_I/1 -> Sum/2
  Sum/1 -> Gain/1
  Gain1/1 -> Gain2/1
  Gain2/1 -> torque/1
  Gain/1 -> Abs/1
  Transfer Fcn/1 -> Gain1/1, Scope1/1
  Product/1 -> Transfer Fcn/1

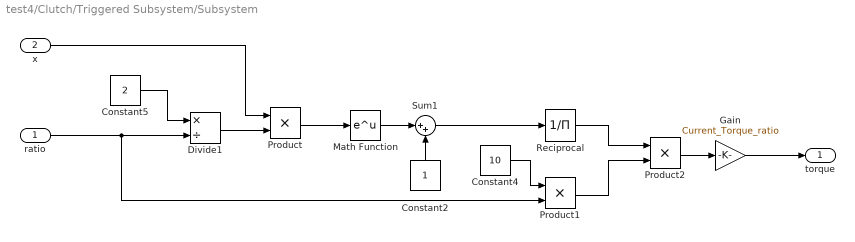
== system test4/Clutch/Triggered Subsystem/Subsystem ==
  ratio : Inport
  x : Inport  Port=2
  Constant2 : Constant
  Constant4 : Constant  Value=10
  Constant5 : Constant  Value=2
  Divide1 : Product  Inputs=*/
  Gain : Gain  Gain=Current_Torque_ratio
  Math Function : Math
  Product : Product
  Product1 : Product
  Product2 : Product
  Reciprocal : Product  Inputs=/
  Sum1 : Sum  Inputs=|++
  torque : Outport
  wires:
  Product1/1 -> Product2/2
  Reciprocal/1 -> Product2/1
  ratio/1 -> Divide1/2, Product1/2
  Constant2/1 -> Sum1/2
  Constant5/1 -> Divide1/1
  Gain/1 -> torque/1
  Product2/1 -> Gain/1
  Product/1 -> Math Function/1
  Constant4/1 -> Product1/1
  x/1 -> Product/1
  Divide1/1 -> Product/2
  Math Function/1 -> Sum1/1
  Sum1/1 -> Reciprocal/1

== matlab function test4/Incremental PID /MATLAB Function ==
  data: Kp input; Pout output; Current_error input; Last_error input
function Pout = fp(Kp, Current_error, Last_error)


Pout = Kp*(Current_error - Last_error);

== matlab function test4/Incremental PID /MATLAB Function2 ==
  data: Kd input; Dout output; Current_error input; Last_error input; Llast_error input
function Dout = fd(Kd, Current_error, Last_error, Llast_error)


Dout = Kd*(Current_error - 2*Last_error + Llast_error);

== matlab function test4/Clutch/Subsystem1/MATLAB Function ==
  data: exp_value input; result output; cur_value input; Range input; interval input
function result = fcn(exp_value, cur_value, Range, interval)

k = -2/Range*log(1 + 1/0.98);

if exp_value/100 == 0.5
    exp_x = 0;
else
    exp_x = real(log(complex((1 - exp_value/100)/(exp_value/100)))/(-k));
end


if cur_value/100 == 0.5
    cur_x = 0;
else
    cur_x = real(log(complex((1 - cur_value/100)/(cur_value/100)))/(-k));
end


differ = exp_x - cur_x;



Left_boundary = 1/(1+ exp(k*(cur_x - interval)));
Right_boundary = 1/(1+ exp(k*(cur_x + interval)));

if (Left_boundary > exp_value)&&(Right_boundary < exp_value)
   
    result = exp_value;

    if (differ < 0)
        result = 1/(1+ exp(k*(cur_x - interval)));
    elseif (differ > 0)
        result = 1/(1+ exp(k*(cur_x + interval)));
    end

    pause(interval);

else
    result = exp_value;
end

== matlab function test4/Incremental PID 1/MATLAB Function ==
  data: Kp input; Pout output; Current_error input; Last_error input
function Pout = fp(Kp, Current_error, Last_error)


Pout = Kp*(Current_error - Last_error);

== matlab function test4/Incremental PID 1/MATLAB Function2 ==
  data: Kd input; Dout output; Current_error input; Last_error input; Llast_error input
function Dout = fd(Kd, Current_error, Last_error, Llast_error)


Dout = Kd*(Current_error - 2*Last_error + Llast_error);

== matlab function test4/Incremental PID 2/MATLAB Function ==
  data: Kp input; Pout output; Current_error input; Last_error input
function Pout = fp(Kp, Current_error, Last_error)


Pout = Kp*(Current_error - Last_error);

== matlab function test4/Incremental PID 2/MATLAB Function2 ==
  data: Kd input; Dout output; Current_error input; Last_error input; Llast_error input
function Dout = fd(Kd, Current_error, Last_error, Llast_error)


Dout = Kd*(Current_error - 2*Last_error + Llast_error);

== matlab function test4/Clutch/Triggered Subsystem/MATLAB Function ==
  data: Exp_Torq input; Fun_Pos output; Output_Torq input; Current_Torq input; range input; step input
function Fun_Pos = fcn(Exp_Torq, Output_Torq,Current_Torq, range, step)
% 
% range = abs(range);
% 
% if ((Exp_Torq ~= Current_Torq) && (isempty(Exp_Torq)))
%     if (abs(Output_Torq - Exp_Torq) >= Step)
%         Fun_Pos = abs((Output_Torq - Current_Torq)/(Exp_Torq - Current_Torq))*range*2 + step;
%     else
%         if Exp_Torq < Current_Torq
%             Fun_Pos = 0
%         else
%             Fun_Pos = range*2;
%         end
%     end
% else
     Fun_Pos = range;
% end

== matlab function test4/Clutch/Triggered Subsystem/MATLAB Function1 ==
  data: Scale_Ratio input; array output; Function_Range input; Sampling_Frequency input; Current_Output input
function array = fcn(Scale_Ratio, Function_Range, Sampling_Frequency, Current_Output)

% if rem(Function_Range*2*Sampling_Frequency,1) == 0
%     Array_Length = Function_Range*2*Sampling_Frequency;
% else
%     Array_Length = Function_Range*2*Sampling_Frequency + 1;
% end

% timer_id = timer ('TimerFcn',output_torque = signal[t],'ExecutionMode','fixedRate','StartDelay',1);
% start(timer_id);
array = 1;

for i = 0 : 0.1 : 2*2
     array = 10*Scale_Ratio/(1 + exp(-3*(i - Function_Range)/Scale_Ratio)) + Current_Output;
end
